simulink library "rewardLibrary"  (R2022b)
settings: Solver=VariableStepAuto  StartTime=0.0  StopTime=10.0  RelTol=1e-3
values from neighbouring files (symbols this model uses):
  accel_vec = (-4:0.5:4)'    [setUpModel.m]
  Ts = 0.1    [setUpMPC.m]
  TsRL = Ts    [setUpRLEnv.m]
  vel_vec = 0:2:20    [setUpModel.m]
undefined symbols (not defined in the file or in its folder): A, B, C, curvature1, D, D_default, DiscIntNeverNeededParam, E, F, gradbp1, k_sigmoid, steer_lim, t_gap, v_set, x_colpen, y_colpen, Z_colpen
libraries: simulink x379, $bdroot x2, mpcadaslib x1
(part 8 of 9)

== system rewardLibrary/Obs // Reward 8-7/Path following ==
  v_err : Inport
  e1 : Inport  Port=2
  e2 : Inport  Port=3
  steer : Inport  Port=4
  accel : Inport  Port=5
  Exp{,1..4} (5 alike) : Math
  Gain1 : Gain  Gain=0.5
  Gain11 : Gain  Gain=-0.1
  Gain12 : Gain  Gain=1.5
  Gain2 : Gain  Gain=0.2
  Gain3 : Gain  Gain=0.1
  Gain4 : Gain  Gain=-0.5
  Gain5 : Gain  Gain=-10
  Gain6 : Gain  Gain=1.5
  Gain8 : Gain  Gain=-0.1
  Gain9 : Gain  Gain=-0.125
  Math Function2 : Math  Operator=square  SignedPower=on
  Square{1..4} (4 alike) : Math  Operator=square  SignedPower=on
  Sum1 : Sum  Inputs=+++++
  Unit Delay : UnitDelay  SampleTime=-1  HasFrameUpgradeWarning=on
  Unit Delay1 : UnitDelay  SampleTime=-1  HasFrameUpgradeWarning=on
  r_pf : Outport  VectorParamsAs1DForOutWhenUnconnected=off
  wires:
  Gain12/1 -> Sum1/1
  Gain6/1 -> Sum1/2
  Gain1/1 -> Sum1/3
  Gain2/1 -> Sum1/4
  Gain3/1 -> Sum1/5
  Exp4/1 -> Gain3/1
  Exp3/1 -> Gain2/1
  Exp2/1 -> Gain1/1
  Exp1/1 -> Gain6/1
  Gain9/1 -> Exp1/1
  Gain4/1 -> Exp2/1
  Gain5/1 -> Exp3/1
  Gain8/1 -> Exp4/1
  Square1/1 -> Gain9/1
  Math Function2/1 -> Gain5/1
  Square3/1 -> Gain8/1
  Unit Delay1/1 -> Square3/1
  Unit Delay/1 -> Math Function2/1  "u_prev"
  e2/1 -> Square2/1
  e1/1 -> Square1/1
  steer/1 -> Unit Delay/1
  Square2/1 -> Gain4/1
  accel/1 -> Unit Delay1/1
  Sum1/1 -> r_pf/1
  v_err/1 -> Square4/1
  Exp/1 -> Gain12/1
  Square4/1 -> Gain11/1
  Gain11/1 -> Exp/1

== system rewardLibrary/Obs // Reward 8-7/Subsystem ==
  v_ego : Inport
  v_ref : Inport  Port=2
  e1 : Inport  Port=3
  e2 : Inport  Port=4
  e1dot : Inport  Port=5
  e2dot : Inport  Port=6
  v_lead : Inport  Port=7
  xgap : Inport  Port=8
  ygap : Inport  Port=9
  Add : Sum  Inputs=+-
  Discrete-Time Integrator1 : DiscreteIntegrator  SampleTime=-1  ICPrevOutput=DiscIntNeverNeededParam  ICPrevScaledInput=DiscIntNeverNeededParam
  Discrete-Time Integrator2 : DiscreteIntegrator  SampleTime=-1  ICPrevOutput=DiscIntNeverNeededParam  ICPrevScaledInput=DiscIntNeverNeededParam
  Discrete-Time Integrator3 : DiscreteIntegrator  SampleTime=-1  ICPrevOutput=DiscIntNeverNeededParam  ICPrevScaledInput=DiscIntNeverNeededParam
  Lateral deviation : Scope
  Mux : Mux  Inputs=12
  obs : Outport  VectorParamsAs1DForOutWhenUnconnected=off
  v_err : Outport  Port=2  VectorParamsAs1DForOutWhenUnconnected=off
  wires:
  v_ref/1 -> Add/1  "d_rel"
  e2dot/1 -> Mux/9
  e1dot/1 -> Mux/8
  Mux/1 -> obs/1
  Discrete-Time Integrator2/1 -> Mux/4  "integral_error"
  e2/1 -> Discrete-Time Integrator3/1, Mux/7
  Discrete-Time Integrator1/1 -> Mux/1  "integral_error"
  e1/1 -> Discrete-Time Integrator2/1, Mux/5, Lateral deviation/1
  v_ego/1 -> Mux/3, Add/2
  Discrete-Time Integrator3/1 -> Mux/6  "integral_error"
  Add/1 -> Discrete-Time Integrator1/1, Mux/2, v_err/1
  v_lead/1 -> Mux/10
  xgap/1 -> Mux/11
  ygap/1 -> Mux/12

== system rewardLibrary/Obs // Reward 8-7/Subsystem2 ==
  v_ego : Inport
  e1 : Inport  Port=2
  e2 : Inport  Port=3
  xgap : Inport  Port=4
  collided : Inport  Port=5
  AND : Logic  IconShape=distinctive  AllPortsSameDT=off  OutDataTypeStr=boolean
  AND1 : Logic  IconShape=distinctive  AllPortsSameDT=off  OutDataTypeStr=boolean
  Abs : Abs  SaturateOnIntegerOverflow=off
  Abs1 : Abs  SaturateOnIntegerOverflow=off
  Compare To Constant : simulink/Logic and Bit Operations/Compare To Constant  relop=>  const=90  OutDataTypeStr=boolean
  Compare To Constant1 : simulink/Logic and Bit Operations/Compare To Constant  relop=>  const=0  OutDataTypeStr=boolean
  Constant : Constant
  Constant3 : Constant  Value=0
  Demux : Demux  Outputs=2
  Detect Rise Positive : simulink/Logic and Bit Operations/Detect Rise Positive  vinit=0  OutDataTypeStr=boolean
  Lateral deviation : simulink/Logic and Bit Operations/Compare To Constant  relop=>  const=8  OutDataTypeStr=boolean
  Logical Operator1 : Logic  Operator=OR  Inputs=3  AllPortsSameDT=off  OutDataTypeStr=boolean
  R2D : Gain  Gain=180/pi
  Relative yaw angle : simulink/Logic and Bit Operations/Compare To Constant  relop=>  const=55  OutDataTypeStr=boolean
  Switch : Switch  Criteria=u2 > Threshold  Threshold=90  SaturateOnIntegerOverflow=off  InputSameDT=off
  Terminator : Terminator
  Velocity : simulink/Logic and Bit Operations/Compare To Constant  relop=<  const=2  OutDataTypeStr=boolean
  Velocity1 : simulink/Logic and Bit Operations/Compare To Constant  relop=<  const=10  OutDataTypeStr=boolean
  fail : Outport  VectorParamsAs1DForOutWhenUnconnected=off
  failCollided : Outport  Port=2  VectorParamsAs1DForOutWhenUnconnected=off
  completeCourse : Outport  Port=3  VectorParamsAs1DForOutWhenUnconnected=off
  overtakeSuccess : Outport  Port=4  VectorParamsAs1DForOutWhenUnconnected=off
  wires:
  Demux/2 -> Compare To Constant/1, Switch/2  "y2"
  [pos2] -> Demux/1
  Demux/1 -> Terminator/1
  Logical Operator1/1 -> fail/1
  Constant3/1 -> Switch/3
  Constant/1 -> Switch/1
  Switch/1 -> completeCourse/1
  AND/1 -> Logical Operator1/3  "spinTurn"
  Relative yaw angle/1 -> AND/2
  R2D/1 -> Relative yaw angle/1
  Abs1/1 -> R2D/1
  e2/1 -> Abs1/1
  Velocity1/1 -> AND/1
  e1/1 -> Abs/1
  Abs/1 -> Lateral deviation/1
  v_ego/1 -> Velocity/1, Velocity1/1
  Lateral deviation/1 -> Logical Operator1/2
  Velocity/1 -> Logical Operator1/1  "tooSlow"
  Compare To Constant/1 -> Detect Rise Positive/1
  Detect Rise Positive/1 -> AND1/1
  xgap/1 -> Compare To Constant1/1
  Compare To Constant1/1 -> AND1/2
  AND1/1 -> overtakeSuccess/1
  collided/1 -> failCollided/1

== system rewardLibrary/Obs // Reward 8-9/Overtaking ==
  ry : Inport
  G : Inport  Port=2
  Add : Sum  Inputs=+-
  Compare To Constant : simulink/Logic and Bit Operations/Compare To Constant  Commented=on  relop=>  const=0  OutDataTypeStr=boolean
  Constant : Constant
  Constant1 : Constant  Value=0
  D : Gain  Gain=2
  F : Gain  Commented=on  Gain=3
  Gain1 : Gain  Gain=2
  Gain6 : Gain  Gain=0.75
  Sigmoid : Subsystem
  Slipstream reward enable : Switch  Criteria=u2 > Threshold  Threshold=-5  SaturateOnIntegerOverflow=off  InputSameDT=off
  Sum1 : Sum  Inputs=+++
  r_ot : Outport  VectorParamsAs1DForOutWhenUnconnected=off
  wires:
  Compare To Constant/1 -> F/1
  F/1 -> Sum1/3
  Constant1/1 -> Slipstream reward enable/1
  Gain6/1 -> Slipstream reward enable/3
  G/1 -> Sigmoid/1(x), Slipstream reward enable/2, Compare To Constant/1
  Add/1 -> D/1
  D/1 -> Sum1/2
  Constant/1 -> Add/2
  Gain1/1 -> Add/1
  Sigmoid/1(sigmoid) -> Gain1/1
  ry/1 -> Gain6/1
  Slipstream reward enable/1 -> Sum1/1
  Sum1/1 -> r_ot/1

== system rewardLibrary/Obs // Reward 8-9/Path following ==
  v_err : Inport
  e1 : Inport  Port=2
  e2 : Inport  Port=3
  steer : Inport  Port=4
  accel : Inport  Port=5
  Exp{,1..4} (5 alike) : Math
  Gain1 : Gain  Gain=0.5
  Gain11 : Gain  Gain=-0.006
  Gain12 : Gain  Gain=4
  Gain2 : Gain  Gain=0.2
  Gain3 : Gain  Gain=0.1
  Gain4 : Gain  Gain=-0.9
  Gain5 : Gain  Gain=-10
  Gain6 : Gain  Gain=1.5
  Gain8 : Gain  Gain=-0.1
  Gain9 : Gain  Gain=-0.125
  Math Function2 : Math  Operator=square  SignedPower=on
  Square{1..4} (4 alike) : Math  Operator=square  SignedPower=on
  Sum1 : Sum  Inputs=+++++
  Unit Delay : UnitDelay  SampleTime=-1  HasFrameUpgradeWarning=on
  Unit Delay1 : UnitDelay  SampleTime=-1  HasFrameUpgradeWarning=on
  r_pf : Outport  VectorParamsAs1DForOutWhenUnconnected=off
  wires:
  Gain11/1 -> Exp/1
  Square4/1 -> Gain11/1
  Exp/1 -> Gain12/1
  v_err/1 -> Square4/1
  Sum1/1 -> r_pf/1
  accel/1 -> Unit Delay1/1
  Square2/1 -> Gain4/1
  steer/1 -> Unit Delay/1
  e1/1 -> Square1/1
  e2/1 -> Square2/1
  Unit Delay/1 -> Math Function2/1  "u_prev"
  Unit Delay1/1 -> Square3/1
  Square3/1 -> Gain8/1
  Math Function2/1 -> Gain5/1
  Square1/1 -> Gain9/1
  Gain8/1 -> Exp4/1
  Gain5/1 -> Exp3/1
  Gain4/1 -> Exp2/1
  Gain9/1 -> Exp1/1
  Exp1/1 -> Gain6/1
  Exp2/1 -> Gain1/1
  Exp3/1 -> Gain2/1
  Exp4/1 -> Gain3/1
  Gain3/1 -> Sum1/5
  Gain2/1 -> Sum1/4
  Gain1/1 -> Sum1/3
  Gain6/1 -> Sum1/2
  Gain12/1 -> Sum1/1

== system rewardLibrary/Obs // Reward 8-9/Subsystem ==
  v_ego : Inport
  v_ref : Inport  Port=2
  e1 : Inport  Port=3
  e2 : Inport  Port=4
  e1dot : Inport  Port=5
  e2dot : Inport  Port=6
  v_lead : Inport  Port=7
  xgap : Inport  Port=8
  ygap : Inport  Port=9
  Add : Sum  Inputs=+-
  Discrete-Time Integrator1 : DiscreteIntegrator  SampleTime=-1  ICPrevOutput=DiscIntNeverNeededParam  ICPrevScaledInput=DiscIntNeverNeededParam
  Discrete-Time Integrator2 : DiscreteIntegrator  SampleTime=-1  ICPrevOutput=DiscIntNeverNeededParam  ICPrevScaledInput=DiscIntNeverNeededParam
  Discrete-Time Integrator3 : DiscreteIntegrator  SampleTime=-1  ICPrevOutput=DiscIntNeverNeededParam  ICPrevScaledInput=DiscIntNeverNeededParam
  Lateral deviation : Scope
  Mux : Mux  Inputs=12
  obs : Outport  VectorParamsAs1DForOutWhenUnconnected=off
  v_err : Outport  Port=2  VectorParamsAs1DForOutWhenUnconnected=off
  wires:
  ygap/1 -> Mux/12
  xgap/1 -> Mux/11
  v_lead/1 -> Mux/10
  Add/1 -> v_err/1, Mux/2, Discrete-Time Integrator1/1
  Discrete-Time Integrator3/1 -> Mux/6  "integral_error"
  v_ego/1 -> Add/2, Mux/3
  e1/1 -> Lateral deviation/1, Mux/5, Discrete-Time Integrator2/1
  Discrete-Time Integrator1/1 -> Mux/1  "integral_error"
  e2/1 -> Mux/7, Discrete-Time Integrator3/1
  Discrete-Time Integrator2/1 -> Mux/4  "integral_error"
  Mux/1 -> obs/1
  e1dot/1 -> Mux/8
  e2dot/1 -> Mux/9
  v_ref/1 -> Add/1  "d_rel"

== system rewardLibrary/Obs // Reward 8-9/Subsystem2 ==
  v_ego : Inport
  e1 : Inport  Port=2
  e2 : Inport  Port=3
  xgap : Inport  Port=4
  collided : Inport  Port=5
  AND : Logic  IconShape=distinctive  AllPortsSameDT=off  OutDataTypeStr=boolean
  AND1 : Logic  IconShape=distinctive  AllPortsSameDT=off  OutDataTypeStr=boolean
  Abs : Abs  SaturateOnIntegerOverflow=off
  Abs1 : Abs  SaturateOnIntegerOverflow=off
  Compare To Constant : simulink/Logic and Bit Operations/Compare To Constant  relop=>  const=90  OutDataTypeStr=boolean
  Compare To Constant1 : simulink/Logic and Bit Operations/Compare To Constant  relop=>  const=0  OutDataTypeStr=boolean
  Constant : Constant
  Constant3 : Constant  Value=0
  Demux : Demux  Outputs=2
  Detect Rise Positive : simulink/Logic and Bit Operations/Detect Rise Positive  vinit=0  OutDataTypeStr=boolean
  Lateral deviation : simulink/Logic and Bit Operations/Compare To Constant  relop=>  const=8  OutDataTypeStr=boolean
  Logical Operator1 : Logic  Operator=OR  Inputs=3  AllPortsSameDT=off  OutDataTypeStr=boolean
  R2D : Gain  Gain=180/pi
  Relative yaw angle : simulink/Logic and Bit Operations/Compare To Constant  relop=>  const=55  OutDataTypeStr=boolean
  Switch : Switch  Criteria=u2 > Threshold  Threshold=90  SaturateOnIntegerOverflow=off  InputSameDT=off
  Terminator : Terminator
  Velocity : simulink/Logic and Bit Operations/Compare To Constant  relop=<  const=2  OutDataTypeStr=boolean
  Velocity1 : simulink/Logic and Bit Operations/Compare To Constant  relop=<  const=10  OutDataTypeStr=boolean
  fail : Outport  VectorParamsAs1DForOutWhenUnconnected=off
  failCollided : Outport  Port=2  VectorParamsAs1DForOutWhenUnconnected=off
  completeCourse : Outport  Port=3  VectorParamsAs1DForOutWhenUnconnected=off
  overtakeSuccess : Outport  Port=4  VectorParamsAs1DForOutWhenUnconnected=off
  wires:
  collided/1 -> failCollided/1
  AND1/1 -> overtakeSuccess/1
  Compare To Constant1/1 -> AND1/2
  xgap/1 -> Compare To Constant1/1
  Detect Rise Positive/1 -> AND1/1
  Compare To Constant/1 -> Detect Rise Positive/1
  Velocity/1 -> Logical Operator1/1  "tooSlow"
  Lateral deviation/1 -> Logical Operator1/2
  v_ego/1 -> Velocity1/1, Velocity/1
  Abs/1 -> Lateral deviation/1
  e1/1 -> Abs/1
  Velocity1/1 -> AND/1
  e2/1 -> Abs1/1
  Abs1/1 -> R2D/1
  R2D/1 -> Relative yaw angle/1
  Relative yaw angle/1 -> AND/2
  AND/1 -> Logical Operator1/3  "spinTurn"
  Switch/1 -> completeCourse/1
  Constant/1 -> Switch/1
  Constant3/1 -> Switch/3
  Logical Operator1/1 -> fail/1
  Demux/1 -> Terminator/1
  [pos2] -> Demux/1
  Demux/2 -> Switch/2, Compare To Constant/1  "y2"

== system rewardLibrary/Obs // Reward 9-1/Overtaking ==
  note: lead
  ry : Inport
  G : Inport  Port=2
  -k : Gain  Gain=-0.4
  Add : Sum
  Add1 : Sum  Inputs=+-
  C : Gain  Gain=0
  Constant : Constant
  Constant1 : Constant  Value=0
  Constant2 : Constant
  D : Gain  Gain=3
  Divide : Product  Inputs=*/
  Exp : Math
  Slipstream reward enable : Switch  Criteria=u2 > Threshold  Threshold=-6.5  SaturateOnIntegerOverflow=off  InputSameDT=off
  Sum1 : Sum
  h : Constant  Value=-2
  r_ot : Outport  VectorParamsAs1DForOutWhenUnconnected=off
  wires:
  Constant1/1 -> Slipstream reward enable/1
  C/1 -> Slipstream reward enable/3
  Divide/1 -> D/1
  ry/1 -> C/1
  Slipstream reward enable/1 -> Sum1/1
  Sum1/1 -> r_ot/1
  D/1 -> Sum1/2
  Exp/1 -> Add/1
  G/1 -> Add1/1, Slipstream reward enable/2
  Constant/1 -> Divide/1
  -k/1 -> Exp/1
  Constant2/1 -> Add/2
  Add/1 -> Divide/2
  Add1/1 -> -k/1
  h/1 -> Add1/2

== system rewardLibrary/Obs // Reward 9-1/Path following ==
  v_err : Inport
  e1 : Inport  Port=2
  e2 : Inport  Port=3
  steer : Inport  Port=4
  accel : Inport  Port=5
  Constant : Constant  Value=0.5
  Exp{,1..4} (5 alike) : Math
  Gain1 : Gain  Gain=0.5
  Gain11 : Gain  Gain=-0.15
  Gain12 : Gain
  Gain2 : Gain  Gain=0.2
  Gain3 : Gain  Gain=0.1
  Gain4 : Gain  Gain=-0.9
  Gain5 : Gain  Gain=-10
  Gain6 : Gain  Gain=1.5
  Gain8 : Gain  Gain=-0.1
  Gain9 : Gain  Gain=-0.06
  Math Function2 : Math  Operator=square  SignedPower=on
  Square{1..4} (4 alike) : Math  Operator=square  SignedPower=on
  Sum1 : Sum  Inputs=++++++
  Unit Delay : UnitDelay  SampleTime=-1  HasFrameUpgradeWarning=on
  Unit Delay1 : UnitDelay  SampleTime=-1  HasFrameUpgradeWarning=on
  r_pf : Outport  VectorParamsAs1DForOutWhenUnconnected=off
  wires:
  Gain11/1 -> Exp/1
  Square4/1 -> Gain11/1
  Exp/1 -> Gain12/1
  v_err/1 -> Square4/1
  Sum1/1 -> r_pf/1
  accel/1 -> Unit Delay1/1
  Square2/1 -> Gain4/1
  steer/1 -> Unit Delay/1
  e1/1 -> Square1/1
  e2/1 -> Square2/1
  Unit Delay/1 -> Math Function2/1  "u_prev"
  Unit Delay1/1 -> Square3/1
  Square3/1 -> Gain8/1
  Math Function2/1 -> Gain5/1
  Square1/1 -> Gain9/1
  Gain8/1 -> Exp4/1
  Gain5/1 -> Exp3/1
  Gain4/1 -> Exp2/1
  Gain9/1 -> Exp1/1
  Exp1/1 -> Gain6/1
  Exp2/1 -> Gain1/1
  Exp3/1 -> Gain2/1
  Exp4/1 -> Gain3/1
  Gain3/1 -> Sum1/5
  Gain2/1 -> Sum1/4
  Gain1/1 -> Sum1/3
  Gain6/1 -> Sum1/2
  Gain12/1 -> Sum1/1
  Constant/1 -> Sum1/6

== system rewardLibrary/Obs // Reward 9-1/Subsystem ==
  v_ego : Inport
  v_ref : Inport  Port=2
  e1 : Inport  Port=3
  e2 : Inport  Port=4
  e1dot : Inport  Port=5
  e2dot : Inport  Port=6
  v_lead : Inport  Port=7
  xgap : Inport  Port=8
  ygap : Inport  Port=9
  Add : Sum  Inputs=+-
  Discrete-Time Integrator1 : DiscreteIntegrator  SampleTime=-1  ICPrevOutput=DiscIntNeverNeededParam  ICPrevScaledInput=DiscIntNeverNeededParam
  Discrete-Time Integrator2 : DiscreteIntegrator  SampleTime=-1  ICPrevOutput=DiscIntNeverNeededParam  ICPrevScaledInput=DiscIntNeverNeededParam
  Discrete-Time Integrator3 : DiscreteIntegrator  SampleTime=-1  ICPrevOutput=DiscIntNeverNeededParam  ICPrevScaledInput=DiscIntNeverNeededParam
  Lateral deviation : Scope
  Mux : Mux  Inputs=12
  obs : Outport  VectorParamsAs1DForOutWhenUnconnected=off
  v_err : Outport  Port=2  VectorParamsAs1DForOutWhenUnconnected=off
  wires:
  ygap/1 -> Mux/12
  xgap/1 -> Mux/11
  v_lead/1 -> Mux/10
  Add/1 -> v_err/1, Mux/2, Discrete-Time Integrator1/1
  Discrete-Time Integrator3/1 -> Mux/6  "integral_error"
  v_ego/1 -> Add/2, Mux/3
  e1/1 -> Lateral deviation/1, Mux/5, Discrete-Time Integrator2/1
  Discrete-Time Integrator1/1 -> Mux/1  "integral_error"
  e2/1 -> Mux/7, Discrete-Time Integrator3/1
  Discrete-Time Integrator2/1 -> Mux/4  "integral_error"
  Mux/1 -> obs/1
  e1dot/1 -> Mux/8
  e2dot/1 -> Mux/9
  v_ref/1 -> Add/1  "d_rel"

== system rewardLibrary/Obs // Reward 9-1/Subsystem2 ==
  v_ego : Inport
  e1 : Inport  Port=2
  e2 : Inport  Port=3
  xgap : Inport  Port=4
  collided : Inport  Port=5
  AND : Logic  IconShape=distinctive  AllPortsSameDT=off  OutDataTypeStr=boolean
  AND1 : Logic  IconShape=distinctive  AllPortsSameDT=off  OutDataTypeStr=boolean
  Abs : Abs  SaturateOnIntegerOverflow=off
  Abs1 : Abs  SaturateOnIntegerOverflow=off
  Compare To Constant : simulink/Logic and Bit Operations/Compare To Constant  relop=>  const=90  OutDataTypeStr=boolean
  Compare To Constant1 : simulink/Logic and Bit Operations/Compare To Constant  relop=>  const=0  OutDataTypeStr=boolean
  Constant : Constant
  Constant3 : Constant  Value=0
  Demux : Demux  Outputs=2
  Detect Rise Positive : simulink/Logic and Bit Operations/Detect Rise Positive  vinit=0  OutDataTypeStr=boolean
  Lateral deviation : simulink/Logic and Bit Operations/Compare To Constant  relop=>  const=8  OutDataTypeStr=boolean
  Logical Operator1 : Logic  Operator=OR  Inputs=3  AllPortsSameDT=off  OutDataTypeStr=boolean
  R2D : Gain  Gain=180/pi
  Relative yaw angle : simulink/Logic and Bit Operations/Compare To Constant  relop=>  const=40  OutDataTypeStr=boolean
  Switch : Switch  Criteria=u2 > Threshold  Threshold=90  SaturateOnIntegerOverflow=off  InputSameDT=off
  Terminator : Terminator
  Velocity : simulink/Logic and Bit Operations/Compare To Constant  relop=<  const=2  OutDataTypeStr=boolean
  Velocity1 : simulink/Logic and Bit Operations/Compare To Constant  relop=<  const=10  OutDataTypeStr=boolean
  fail : Outport  VectorParamsAs1DForOutWhenUnconnected=off
  failCollided : Outport  Port=2  VectorParamsAs1DForOutWhenUnconnected=off
  completeCourse : Outport  Port=3  VectorParamsAs1DForOutWhenUnconnected=off
  overtakeSuccess : Outport  Port=4  VectorParamsAs1DForOutWhenUnconnected=off
  wires:
  collided/1 -> failCollided/1
  AND1/1 -> overtakeSuccess/1
  Compare To Constant1/1 -> AND1/2
  xgap/1 -> Compare To Constant1/1
  Detect Rise Positive/1 -> AND1/1
  Compare To Constant/1 -> Detect Rise Positive/1
  Velocity/1 -> Logical Operator1/1  "tooSlow"
  Lateral deviation/1 -> Logical Operator1/2
  v_ego/1 -> Velocity1/1, Velocity/1
  Abs/1 -> Lateral deviation/1
  e1/1 -> Abs/1
  Velocity1/1 -> AND/1
  e2/1 -> Abs1/1
  Abs1/1 -> R2D/1
  R2D/1 -> Relative yaw angle/1
  Relative yaw angle/1 -> AND/2
  AND/1 -> Logical Operator1/3  "spinTurn"
  Switch/1 -> completeCourse/1
  Constant/1 -> Switch/1
  Constant3/1 -> Switch/3
  Logical Operator1/1 -> fail/1
  Demux/1 -> Terminator/1
  [pos2] -> Demux/1
  Demux/2 -> Switch/2, Compare To Constant/1  "y2"

== system rewardLibrary/Obs // Reward 9-2/Overtaking ==
  note: Overtake on right sigmoid
  note: Overtaking reward sigmoid
  ry : Inport
  xgap : Inport  Port=2
  ygap : Inport  Port=3
  -k : Gain  Gain=-0.4
  -k1 : Gain  Gain=-3
  Add : Sum
  Add1 : Sum  Inputs=+-
  Add2 : Sum
  C : Gain  Gain=0
  Constant{,2..4} (4 alike) : Constant
  Constant1 : Constant  Value=0
  Constant5 : Constant  Value=0
  D : Gain  Gain=3
  Divide : Product  Inputs=*/
  Divide1 : Product  Inputs=*/
  Exp : Math
  Exp1 : Math
  G : Gain
  Slipstream reward enable : Switch  Criteria=u2 > Threshold  Threshold=-6.5  SaturateOnIntegerOverflow=off  InputSameDT=off
  Slipstream reward enable1 : Switch  Criteria=u2 > Threshold  SaturateOnIntegerOverflow=off  InputSameDT=off
  Sum1 : Sum  Inputs=+++
  h : Constant  Value=-2
  r_ot : Outport  VectorParamsAs1DForOutWhenUnconnected=off
  wires:
  Constant1/1 -> Slipstream reward enable/1
  C/1 -> Slipstream reward enable/3
  Divide/1 -> D/1
  ry/1 -> C/1
  Slipstream reward enable/1 -> Sum1/1
  Sum1/1 -> r_ot/1
  D/1 -> Sum1/2
  Exp/1 -> Add/1
  xgap/1 -> Slipstream reward enable/2, Slipstream reward enable1/2, Add1/1
  Constant/1 -> Divide/1
  -k/1 -> Exp/1
  Constant2/1 -> Add/2
  Add/1 -> Divide/2
  Add1/1 -> -k/1
  h/1 -> Add1/2
  Constant4/1 -> Add2/2
  Add2/1 -> Divide1/2
  -k1/1 -> Exp1/1
  Exp1/1 -> Add2/1
  Constant3/1 -> Divide1/1
  Divide1/1 -> G/1
  G/1 -> Sum1/3
  ygap/1 -> Slipstream reward enable1/3
  Constant5/1 -> Slipstream reward enable1/1
  Slipstream reward enable1/1 -> -k1/1

== system rewardLibrary/Obs // Reward 9-2/Path following ==
  v_err : Inport
  e1 : Inport  Port=2
  e2 : Inport  Port=3
  steer : Inport  Port=4
  accel : Inport  Port=5
  Constant : Constant  Commented=on  Value=0.5
  Exp{,1..4} (5 alike) : Math
  Gain1 : Gain  Gain=0.5
  Gain11 : Gain  Gain=-0.15
  Gain12 : Gain
  Gain2 : Gain  Gain=0.2
  Gain3 : Gain  Gain=0.1
  Gain4 : Gain  Gain=-0.9
  Gain5 : Gain  Gain=-10
  Gain6 : Gain  Gain=1.5
  Gain8 : Gain  Gain=-0.1
  Gain9 : Gain  Gain=-0.06
  Math Function2 : Math  Operator=square  SignedPower=on
  Square{1..4} (4 alike) : Math  Operator=square  SignedPower=on
  Sum1 : Sum  Inputs=++++++
  Unit Delay : UnitDelay  SampleTime=-1  HasFrameUpgradeWarning=on
  Unit Delay1 : UnitDelay  SampleTime=-1  HasFrameUpgradeWarning=on
  r_pf : Outport  VectorParamsAs1DForOutWhenUnconnected=off
  wires:
  Gain11/1 -> Exp/1
  Square4/1 -> Gain11/1
  Exp/1 -> Gain12/1
  v_err/1 -> Square4/1
  Sum1/1 -> r_pf/1
  accel/1 -> Unit Delay1/1
  Square2/1 -> Gain4/1
  steer/1 -> Unit Delay/1
  e1/1 -> Square1/1
  e2/1 -> Square2/1
  Unit Delay/1 -> Math Function2/1  "u_prev"
  Unit Delay1/1 -> Square3/1
  Square3/1 -> Gain8/1
  Math Function2/1 -> Gain5/1
  Square1/1 -> Gain9/1
  Gain8/1 -> Exp4/1
  Gain5/1 -> Exp3/1
  Gain4/1 -> Exp2/1
  Gain9/1 -> Exp1/1
  Exp1/1 -> Gain6/1
  Exp2/1 -> Gain1/1
  Exp3/1 -> Gain2/1
  Exp4/1 -> Gain3/1
  Gain3/1 -> Sum1/5
  Gain2/1 -> Sum1/4
  Gain1/1 -> Sum1/3
  Gain6/1 -> Sum1/2
  Gain12/1 -> Sum1/1
  Constant/1 -> Sum1/6

== system rewardLibrary/Obs // Reward 9-2/Subsystem ==
  v_ego : Inport
  v_ref : Inport  Port=2
  e1 : Inport  Port=3
  e2 : Inport  Port=4
  e1dot : Inport  Port=5
  e2dot : Inport  Port=6
  v_lead : Inport  Port=7
  xgap : Inport  Port=8
  ygap : Inport  Port=9
  Add : Sum  Inputs=+-
  Discrete-Time Integrator1 : DiscreteIntegrator  SampleTime=-1  ICPrevOutput=DiscIntNeverNeededParam  ICPrevScaledInput=DiscIntNeverNeededParam
  Discrete-Time Integrator2 : DiscreteIntegrator  SampleTime=-1  ICPrevOutput=DiscIntNeverNeededParam  ICPrevScaledInput=DiscIntNeverNeededParam
  Discrete-Time Integrator3 : DiscreteIntegrator  SampleTime=-1  ICPrevOutput=DiscIntNeverNeededParam  ICPrevScaledInput=DiscIntNeverNeededParam
  Lateral deviation : Scope
  Mux : Mux  Inputs=12
  obs : Outport  VectorParamsAs1DForOutWhenUnconnected=off
  v_err : Outport  Port=2  VectorParamsAs1DForOutWhenUnconnected=off
  wires:
  ygap/1 -> Mux/12
  xgap/1 -> Mux/11
  v_lead/1 -> Mux/10
  Add/1 -> v_err/1, Mux/2, Discrete-Time Integrator1/1
  Discrete-Time Integrator3/1 -> Mux/6  "integral_error"
  v_ego/1 -> Add/2, Mux/3
  e1/1 -> Lateral deviation/1, Mux/5, Discrete-Time Integrator2/1
  Discrete-Time Integrator1/1 -> Mux/1  "integral_error"
  e2/1 -> Mux/7, Discrete-Time Integrator3/1
  Discrete-Time Integrator2/1 -> Mux/4  "integral_error"
  Mux/1 -> obs/1
  e1dot/1 -> Mux/8
  e2dot/1 -> Mux/9
  v_ref/1 -> Add/1  "d_rel"

== system rewardLibrary/Obs // Reward 9-2/Subsystem2 ==
  v_ego : Inport
  e1 : Inport  Port=2
  e2 : Inport  Port=3
  xgap : Inport  Port=4
  collided : Inport  Port=5
  AND : Logic  IconShape=distinctive  AllPortsSameDT=off  OutDataTypeStr=boolean
  AND1 : Logic  IconShape=distinctive  AllPortsSameDT=off  OutDataTypeStr=boolean
  Abs : Abs  SaturateOnIntegerOverflow=off
  Abs1 : Abs  SaturateOnIntegerOverflow=off
  Compare To Constant : simulink/Logic and Bit Operations/Compare To Constant  relop=>  const=90  OutDataTypeStr=boolean
  Compare To Constant1 : simulink/Logic and Bit Operations/Compare To Constant  relop=>  const=0  OutDataTypeStr=boolean
  Constant : Constant
  Constant3 : Constant  Value=0
  Demux : Demux  Outputs=2
  Detect Rise Positive : simulink/Logic and Bit Operations/Detect Rise Positive  vinit=0  OutDataTypeStr=boolean
  Lateral deviation : simulink/Logic and Bit Operations/Compare To Constant  relop=>  const=8  OutDataTypeStr=boolean
  Logical Operator1 : Logic  Operator=OR  Inputs=3  AllPortsSameDT=off  OutDataTypeStr=boolean
  R2D : Gain  Gain=180/pi
  Relative yaw angle : simulink/Logic and Bit Operations/Compare To Constant  relop=>  const=40  OutDataTypeStr=boolean
  Switch : Switch  Criteria=u2 > Threshold  Threshold=90  SaturateOnIntegerOverflow=off  InputSameDT=off
  Terminator : Terminator
  Velocity : simulink/Logic and Bit Operations/Compare To Constant  relop=<  const=2  OutDataTypeStr=boolean
  Velocity1 : simulink/Logic and Bit Operations/Compare To Constant  relop=<  const=10  OutDataTypeStr=boolean
  fail : Outport  VectorParamsAs1DForOutWhenUnconnected=off
  failCollided : Outport  Port=2  VectorParamsAs1DForOutWhenUnconnected=off
  completeCourse : Outport  Port=3  VectorParamsAs1DForOutWhenUnconnected=off
  overtakeSuccess : Outport  Port=4  VectorParamsAs1DForOutWhenUnconnected=off
  wires:
  collided/1 -> failCollided/1
  AND1/1 -> overtakeSuccess/1
  Compare To Constant1/1 -> AND1/2
  xgap/1 -> Compare To Constant1/1
  Detect Rise Positive/1 -> AND1/1
  Compare To Constant/1 -> Detect Rise Positive/1
  Velocity/1 -> Logical Operator1/1  "tooSlow"
  Lateral deviation/1 -> Logical Operator1/2
  v_ego/1 -> Velocity1/1, Velocity/1
  Abs/1 -> Lateral deviation/1
  e1/1 -> Abs/1
  Velocity1/1 -> AND/1
  e2/1 -> Abs1/1
  Abs1/1 -> R2D/1
  R2D/1 -> Relative yaw angle/1
  Relative yaw angle/1 -> AND/2
  AND/1 -> Logical Operator1/3  "spinTurn"
  Switch/1 -> completeCourse/1
  Constant/1 -> Switch/1
  Constant3/1 -> Switch/3
  Logical Operator1/1 -> fail/1
  Demux/1 -> Terminator/1
  [pos2] -> Demux/1
  Demux/2 -> Switch/2, Compare To Constant/1  "y2"

== system rewardLibrary/Obs // Reward 9-3/Overtaking ==
  note: Overtake on right sigmoid
  note: Overtaking reward sigmoid
  ry : Inport
  xgap : Inport  Port=2
  ygap : Inport  Port=3
  -k_D : Gain  Gain=-0.4
  -k_G : Gain  Gain=-1.2
  Add : Sum
  Add1 : Sum  Inputs=+-
  Add2 : Sum
  C : Gain  Gain=0
  Constant{,2..4} (4 alike) : Constant
  Constant1 : Constant  Value=0
  D : Gain  Gain=3
  Divide : Product  Inputs=*/
  Divide1 : Product  Inputs=*/
  Exp : Math
  Exp1 : Math
  G : Gain  Gain=0.5
  G1 : Constant  Value=0.5
  Memory : Memory
  Slipstream reward enable : Switch  Criteria=u2 > Threshold  Threshold=-6.5  SaturateOnIntegerOverflow=off  InputSameDT=off
  Subsystem : Subsystem  Commented=on
  Sum1 : Sum  Inputs=+++
  h : Constant  Value=-2
  switch2 : Switch  Criteria=u2 > Threshold  SaturateOnIntegerOverflow=off  InputSameDT=off
  r_ot : Outport  VectorParamsAs1DForOutWhenUnconnected=off
  wires:
  Constant1/1 -> Slipstream reward enable/1
  C/1 -> Slipstream reward enable/3
  Divide/1 -> D/1
  ry/1 -> C/1
  Slipstream reward enable/1 -> Sum1/1
  Sum1/1 -> r_ot/1
  D/1 -> Sum1/2
  Exp/1 -> Add/1
  Constant/1 -> Divide/1
  -k_D/1 -> Exp/1
  Constant2/1 -> Add/2
  Add/1 -> Divide/2
  Add1/1 -> -k_D/1
  h/1 -> Add1/2
  Constant4/1 -> Add2/2
  Add2/1 -> Divide1/2
  -k_G/1 -> Exp1/1
  Exp1/1 -> Add2/1
  Constant3/1 -> Divide1/1
  Divide1/1 -> G/1
  ygap/1 -> -k_G/1
  xgap/1 -> Slipstream reward enable/2, switch2/2, Add1/1
  G1/1 -> switch2/1
  G/1 -> switch2/3
  switch2/1 -> Sum1/3

== system rewardLibrary/Obs // Reward 9-3/Path following ==
  v_err : Inport
  e1 : Inport  Port=2
  e2 : Inport  Port=3
  steer : Inport  Port=4
  accel : Inport  Port=5
  Constant : Constant  Commented=on  Value=0.5
  Exp{,1..4} (5 alike) : Math
  Gain1 : Gain  Gain=0.5
  Gain11 : Gain  Gain=-0.15
  Gain12 : Gain
  Gain2 : Gain  Gain=0.2
  Gain3 : Gain  Gain=0.1
  Gain4 : Gain  Gain=-0.9
  Gain5 : Gain  Gain=-10
  Gain6 : Gain  Gain=1.5
  Gain8 : Gain  Gain=-0.1
  Gain9 : Gain  Gain=-0.06
  Math Function2 : Math  Operator=square  SignedPower=on
  Square{1..4} (4 alike) : Math  Operator=square  SignedPower=on
  Sum1 : Sum  Inputs=++++++
  Unit Delay : UnitDelay  SampleTime=-1  HasFrameUpgradeWarning=on
  Unit Delay1 : UnitDelay  SampleTime=-1  HasFrameUpgradeWarning=on
  r_pf : Outport  VectorParamsAs1DForOutWhenUnconnected=off
  wires:
  Gain11/1 -> Exp/1
  Square4/1 -> Gain11/1
  Exp/1 -> Gain12/1
  v_err/1 -> Square4/1
  Sum1/1 -> r_pf/1
  accel/1 -> Unit Delay1/1
  Square2/1 -> Gain4/1
  steer/1 -> Unit Delay/1
  e1/1 -> Square1/1
  e2/1 -> Square2/1
  Unit Delay/1 -> Math Function2/1  "u_prev"
  Unit Delay1/1 -> Square3/1
  Square3/1 -> Gain8/1
  Math Function2/1 -> Gain5/1
  Square1/1 -> Gain9/1
  Gain8/1 -> Exp4/1
  Gain5/1 -> Exp3/1
  Gain4/1 -> Exp2/1
  Gain9/1 -> Exp1/1
  Exp1/1 -> Gain6/1
  Exp2/1 -> Gain1/1
  Exp3/1 -> Gain2/1
  Exp4/1 -> Gain3/1
  Gain3/1 -> Sum1/5
  Gain2/1 -> Sum1/4
  Gain1/1 -> Sum1/3
  Gain6/1 -> Sum1/2
  Gain12/1 -> Sum1/1
  Constant/1 -> Sum1/6

== system rewardLibrary/Obs // Reward 9-3/Subsystem ==
  v_ego : Inport
  v_ref : Inport  Port=2
  e1 : Inport  Port=3
  e2 : Inport  Port=4
  e1dot : Inport  Port=5
  e2dot : Inport  Port=6
  v_lead : Inport  Port=7
  xgap : Inport  Port=8
  ygap : Inport  Port=9
  Add : Sum  Inputs=+-
  Discrete-Time Integrator1 : DiscreteIntegrator  SampleTime=-1  ICPrevOutput=DiscIntNeverNeededParam  ICPrevScaledInput=DiscIntNeverNeededParam
  Discrete-Time Integrator2 : DiscreteIntegrator  SampleTime=-1  ICPrevOutput=DiscIntNeverNeededParam  ICPrevScaledInput=DiscIntNeverNeededParam
  Discrete-Time Integrator3 : DiscreteIntegrator  SampleTime=-1  ICPrevOutput=DiscIntNeverNeededParam  ICPrevScaledInput=DiscIntNeverNeededParam
  Lateral deviation : Scope
  Mux : Mux  Inputs=12
  obs : Outport  VectorParamsAs1DForOutWhenUnconnected=off
  v_err : Outport  Port=2  VectorParamsAs1DForOutWhenUnconnected=off
  wires:
  ygap/1 -> Mux/12
  xgap/1 -> Mux/11
  v_lead/1 -> Mux/10
  Add/1 -> v_err/1, Mux/2, Discrete-Time Integrator1/1
  Discrete-Time Integrator3/1 -> Mux/6  "integral_error"
  v_ego/1 -> Add/2, Mux/3
  e1/1 -> Lateral deviation/1, Mux/5, Discrete-Time Integrator2/1
  Discrete-Time Integrator1/1 -> Mux/1  "integral_error"
  e2/1 -> Mux/7, Discrete-Time Integrator3/1
  Discrete-Time Integrator2/1 -> Mux/4  "integral_error"
  Mux/1 -> obs/1
  e1dot/1 -> Mux/8
  e2dot/1 -> Mux/9
  v_ref/1 -> Add/1  "d_rel"

== system rewardLibrary/Obs // Reward 9-3/Subsystem2 ==
  v_ego : Inport
  e1 : Inport  Port=2
  e2 : Inport  Port=3
  xgap : Inport  Port=4
  collided : Inport  Port=5
  AND : Logic  IconShape=distinctive  AllPortsSameDT=off  OutDataTypeStr=boolean
  AND1 : Logic  IconShape=distinctive  AllPortsSameDT=off  OutDataTypeStr=boolean
  Abs : Abs  SaturateOnIntegerOverflow=off
  Abs1 : Abs  SaturateOnIntegerOverflow=off
  Compare To Constant : simulink/Logic and Bit Operations/Compare To Constant  relop=>  const=90  OutDataTypeStr=boolean
  Compare To Constant1 : simulink/Logic and Bit Operations/Compare To Constant  relop=>  const=0  OutDataTypeStr=boolean
  Constant : Constant
  Constant3 : Constant  Value=0
  Demux : Demux  Outputs=2
  Detect Rise Positive : simulink/Logic and Bit Operations/Detect Rise Positive  vinit=0  OutDataTypeStr=boolean
  Lateral deviation : simulink/Logic and Bit Operations/Compare To Constant  relop=>  const=8  OutDataTypeStr=boolean
  Logical Operator1 : Logic  Operator=OR  Inputs=3  AllPortsSameDT=off  OutDataTypeStr=boolean
  R2D : Gain  Gain=180/pi
  Relative yaw angle : simulink/Logic and Bit Operations/Compare To Constant  relop=>  const=40  OutDataTypeStr=boolean
  Switch : Switch  Criteria=u2 > Threshold  Threshold=90  SaturateOnIntegerOverflow=off  InputSameDT=off
  Terminator : Terminator
  Velocity : simulink/Logic and Bit Operations/Compare To Constant  relop=<  const=2  OutDataTypeStr=boolean
  Velocity1 : simulink/Logic and Bit Operations/Compare To Constant  relop=<  const=10  OutDataTypeStr=boolean
  fail : Outport  VectorParamsAs1DForOutWhenUnconnected=off
  failCollided : Outport  Port=2  VectorParamsAs1DForOutWhenUnconnected=off
  completeCourse : Outport  Port=3  VectorParamsAs1DForOutWhenUnconnected=off
  overtakeSuccess : Outport  Port=4  VectorParamsAs1DForOutWhenUnconnected=off
  wires:
  collided/1 -> failCollided/1
  AND1/1 -> overtakeSuccess/1
  Compare To Constant1/1 -> AND1/2
  xgap/1 -> Compare To Constant1/1
  Detect Rise Positive/1 -> AND1/1
  Compare To Constant/1 -> Detect Rise Positive/1
  Velocity/1 -> Logical Operator1/1  "tooSlow"
  Lateral deviation/1 -> Logical Operator1/2
  v_ego/1 -> Velocity1/1, Velocity/1
  Abs/1 -> Lateral deviation/1
  e1/1 -> Abs/1
  Velocity1/1 -> AND/1
  e2/1 -> Abs1/1
  Abs1/1 -> R2D/1
  R2D/1 -> Relative yaw angle/1
  Relative yaw angle/1 -> AND/2
  AND/1 -> Logical Operator1/3  "spinTurn"
  Switch/1 -> completeCourse/1
  Constant/1 -> Switch/1
  Constant3/1 -> Switch/3
  Logical Operator1/1 -> fail/1
  Demux/1 -> Terminator/1
  [pos2] -> Demux/1
  Demux/2 -> Switch/2, Compare To Constant/1  "y2"

== system rewardLibrary/Obs // Reward 9-4/Overtaking ==
  note: Overtake on right sigmoid
  note: Overtaking reward sigmoid
  ry : Inport
  xgap : Inport  Port=2
  ygap : Inport  Port=3
  -k_D : Gain  Gain=-0.4
  -k_G : Gain  Gain=-1.2
  Add : Sum
  Add1 : Sum  Inputs=+-
  Add2 : Sum
  C : Gain  Gain=0
  Constant{,2..4} (4 alike) : Constant
  Constant1 : Constant  Value=0
  D : Gain  Gain=9
  Divide : Product  Inputs=*/
  Divide1 : Product  Inputs=*/
  Exp : Math
  Exp1 : Math
  G : Gain  Gain=0.25
  G1 : Constant  Value=0.25
  Memory : Memory
  Slipstream reward enable : Switch  Criteria=u2 > Threshold  Threshold=-6.5  SaturateOnIntegerOverflow=off  InputSameDT=off
  Sum1 : Sum  Inputs=+++
  h : Constant  Value=-2
  switch2 : Switch  Criteria=u2 > Threshold  SaturateOnIntegerOverflow=off  InputSameDT=off
  r_ot : Outport  VectorParamsAs1DForOutWhenUnconnected=off
  wires:
  Constant1/1 -> Slipstream reward enable/1
  C/1 -> Slipstream reward enable/3
  Divide/1 -> D/1
  ry/1 -> C/1
  Slipstream reward enable/1 -> Sum1/1
  Sum1/1 -> r_ot/1
  D/1 -> Sum1/2
  Exp/1 -> Add/1
  Constant/1 -> Divide/1
  -k_D/1 -> Exp/1
  Constant2/1 -> Add/2
  Add/1 -> Divide/2
  Add1/1 -> -k_D/1
  h/1 -> Add1/2
  Constant4/1 -> Add2/2
  Add2/1 -> Divide1/2
  -k_G/1 -> Exp1/1
  Exp1/1 -> Add2/1
  Constant3/1 -> Divide1/1
  Divide1/1 -> G/1
  ygap/1 -> -k_G/1
  xgap/1 -> Slipstream reward enable/2, switch2/2, Add1/1
  G1/1 -> switch2/1
  G/1 -> switch2/3
  switch2/1 -> Sum1/3

== system rewardLibrary/Obs // Reward 9-4/Path following ==
  v_err : Inport
  e1 : Inport  Port=2
  e2 : Inport  Port=3
  steer : Inport  Port=4
  accel : Inport  Port=5
  Constant : Constant  Commented=on  Value=0.5
  Exp{,1..4} (5 alike) : Math
  Gain1 : Gain  Gain=0.5
  Gain11 : Gain  Gain=-0.15
  Gain12 : Gain
  Gain2 : Gain  Gain=0.2
  Gain3 : Gain  Gain=0.1
  Gain4 : Gain  Gain=-0.9
  Gain5 : Gain  Gain=-10
  Gain6 : Gain  Gain=1.5
  Gain8 : Gain  Gain=-0.1
  Gain9 : Gain  Gain=-0.06
  Math Function2 : Math  Operator=square  SignedPower=on
  Square{1..4} (4 alike) : Math  Operator=square  SignedPower=on
  Sum1 : Sum  Inputs=++++++
  Unit Delay : UnitDelay  SampleTime=-1  HasFrameUpgradeWarning=on
  Unit Delay1 : UnitDelay  SampleTime=-1  HasFrameUpgradeWarning=on
  r_pf : Outport  VectorParamsAs1DForOutWhenUnconnected=off
  wires:
  Gain11/1 -> Exp/1
  Square4/1 -> Gain11/1
  Exp/1 -> Gain12/1
  v_err/1 -> Square4/1
  Sum1/1 -> r_pf/1
  accel/1 -> Unit Delay1/1
  Square2/1 -> Gain4/1
  steer/1 -> Unit Delay/1
  e1/1 -> Square1/1
  e2/1 -> Square2/1
  Unit Delay/1 -> Math Function2/1  "u_prev"
  Unit Delay1/1 -> Square3/1
  Square3/1 -> Gain8/1
  Math Function2/1 -> Gain5/1
  Square1/1 -> Gain9/1
  Gain8/1 -> Exp4/1
  Gain5/1 -> Exp3/1
  Gain4/1 -> Exp2/1
  Gain9/1 -> Exp1/1
  Exp1/1 -> Gain6/1
  Exp2/1 -> Gain1/1
  Exp3/1 -> Gain2/1
  Exp4/1 -> Gain3/1
  Gain3/1 -> Sum1/5
  Gain2/1 -> Sum1/4
  Gain1/1 -> Sum1/3
  Gain6/1 -> Sum1/2
  Gain12/1 -> Sum1/1
  Constant/1 -> Sum1/6

== system rewardLibrary/Obs // Reward 9-4/Subsystem ==
  v_ego : Inport
  v_ref : Inport  Port=2
  e1 : Inport  Port=3
  e2 : Inport  Port=4
  e1dot : Inport  Port=5
  e2dot : Inport  Port=6
  v_lead : Inport  Port=7
  xgap : Inport  Port=8
  ygap : Inport  Port=9
  Add : Sum  Inputs=+-
  Discrete-Time Integrator1 : DiscreteIntegrator  SampleTime=-1  ICPrevOutput=DiscIntNeverNeededParam  ICPrevScaledInput=DiscIntNeverNeededParam
  Discrete-Time Integrator2 : DiscreteIntegrator  SampleTime=-1  ICPrevOutput=DiscIntNeverNeededParam  ICPrevScaledInput=DiscIntNeverNeededParam
  Discrete-Time Integrator3 : DiscreteIntegrator  SampleTime=-1  ICPrevOutput=DiscIntNeverNeededParam  ICPrevScaledInput=DiscIntNeverNeededParam
  Lateral deviation : Scope
  Mux : Mux  Inputs=12
  obs : Outport  VectorParamsAs1DForOutWhenUnconnected=off
  v_err : Outport  Port=2  VectorParamsAs1DForOutWhenUnconnected=off
  wires:
  ygap/1 -> Mux/12
  xgap/1 -> Mux/11
  v_lead/1 -> Mux/10
  Add/1 -> v_err/1, Mux/2, Discrete-Time Integrator1/1
  Discrete-Time Integrator3/1 -> Mux/6  "integral_error"
  v_ego/1 -> Add/2, Mux/3
  e1/1 -> Lateral deviation/1, Mux/5, Discrete-Time Integrator2/1
  Discrete-Time Integrator1/1 -> Mux/1  "integral_error"
  e2/1 -> Mux/7, Discrete-Time Integrator3/1
  Discrete-Time Integrator2/1 -> Mux/4  "integral_error"
  Mux/1 -> obs/1
  e1dot/1 -> Mux/8
  e2dot/1 -> Mux/9
  v_ref/1 -> Add/1  "d_rel"

== system rewardLibrary/Obs // Reward 9-4/Subsystem2 ==
  v_ego : Inport
  e1 : Inport  Port=2
  e2 : Inport  Port=3
  xgap : Inport  Port=4
  collided : Inport  Port=5
  AND : Logic  IconShape=distinctive  AllPortsSameDT=off  OutDataTypeStr=boolean
  AND1 : Logic  IconShape=distinctive  AllPortsSameDT=off  OutDataTypeStr=boolean
  Abs : Abs  SaturateOnIntegerOverflow=off
  Abs1 : Abs  SaturateOnIntegerOverflow=off
  Compare To Constant : simulink/Logic and Bit Operations/Compare To Constant  relop=>  const=90  OutDataTypeStr=boolean
  Compare To Constant1 : simulink/Logic and Bit Operations/Compare To Constant  relop=>  const=0  OutDataTypeStr=boolean
  Constant : Constant
  Constant3 : Constant  Value=0
  Demux : Demux  Outputs=2
  Detect Rise Positive : simulink/Logic and Bit Operations/Detect Rise Positive  vinit=0  OutDataTypeStr=boolean
  Lateral deviation : simulink/Logic and Bit Operations/Compare To Constant  relop=>  const=8  OutDataTypeStr=boolean
  Logical Operator1 : Logic  Operator=OR  Inputs=3  AllPortsSameDT=off  OutDataTypeStr=boolean
  R2D : Gain  Gain=180/pi
  Relative yaw angle : simulink/Logic and Bit Operations/Compare To Constant  relop=>  const=30  OutDataTypeStr=boolean
  Switch : Switch  Criteria=u2 > Threshold  Threshold=90  SaturateOnIntegerOverflow=off  InputSameDT=off
  Terminator : Terminator
  Velocity : simulink/Logic and Bit Operations/Compare To Constant  relop=<  const=2  OutDataTypeStr=boolean
  Velocity1 : simulink/Logic and Bit Operations/Compare To Constant  relop=<  const=10  OutDataTypeStr=boolean
  fail : Outport  VectorParamsAs1DForOutWhenUnconnected=off
  failCollided : Outport  Port=2  VectorParamsAs1DForOutWhenUnconnected=off
  completeCourse : Outport  Port=3  VectorParamsAs1DForOutWhenUnconnected=off
  overtakeSuccess : Outport  Port=4  VectorParamsAs1DForOutWhenUnconnected=off
  wires:
  collided/1 -> failCollided/1
  AND1/1 -> overtakeSuccess/1
  Compare To Constant1/1 -> AND1/2
  xgap/1 -> Compare To Constant1/1
  Detect Rise Positive/1 -> AND1/1
  Compare To Constant/1 -> Detect Rise Positive/1
  Velocity/1 -> Logical Operator1/1  "tooSlow"
  Lateral deviation/1 -> Logical Operator1/2
  v_ego/1 -> Velocity1/1, Velocity/1
  Abs/1 -> Lateral deviation/1
  e1/1 -> Abs/1
  Velocity1/1 -> AND/1
  e2/1 -> Abs1/1
  Abs1/1 -> R2D/1
  R2D/1 -> Relative yaw angle/1
  Relative yaw angle/1 -> AND/2
  AND/1 -> Logical Operator1/3  "spinTurn"
  Switch/1 -> completeCourse/1
  Constant/1 -> Switch/1
  Constant3/1 -> Switch/3
  Logical Operator1/1 -> fail/1
  Demux/1 -> Terminator/1
  [pos2] -> Demux/1
  Demux/2 -> Switch/2, Compare To Constant/1  "y2"

== system rewardLibrary/Obs // Reward 9-5/Overtaking ==
  note: Overtake on right sigmoid
  note: Overtaking reward sigmoid
  ry : Inport
  xgap : Inport  Port=2
  ygap : Inport  Port=3
  -k_D : Gain  Gain=-0.4
  -k_G : Gain  Gain=-1.2
  Add : Sum
  Add1 : Sum  Inputs=+-
  Add2 : Sum
  C : Gain  Gain=0
  Constant{,2..4} (4 alike) : Constant
  Constant1 : Constant  Value=0
  D : Gain  Gain=4.25
  Divide : Product  Inputs=*/
  Divide1 : Product  Inputs=*/
  Exp : Math
  Exp1 : Math
  G : Gain  Gain=0.25
  G1 : Constant  Value=0.25
  Slipstream reward enable : Switch  Criteria=u2 > Threshold  Threshold=-6.5  SaturateOnIntegerOverflow=off  InputSameDT=off
  Sum1 : Sum  Inputs=+++
  h : Constant  Value=-2
  switch2 : Switch  Criteria=u2 > Threshold  SaturateOnIntegerOverflow=off  InputSameDT=off
  r_ot : Outport  VectorParamsAs1DForOutWhenUnconnected=off
  wires:
  Constant1/1 -> Slipstream reward enable/1
  C/1 -> Slipstream reward enable/3
  Divide/1 -> D/1
  ry/1 -> C/1
  Slipstream reward enable/1 -> Sum1/1
  Sum1/1 -> r_ot/1
  D/1 -> Sum1/2
  Exp/1 -> Add/1
  Constant/1 -> Divide/1
  -k_D/1 -> Exp/1
  Constant2/1 -> Add/2
  Add/1 -> Divide/2
  Add1/1 -> -k_D/1
  h/1 -> Add1/2
  Constant4/1 -> Add2/2
  Add2/1 -> Divide1/2
  -k_G/1 -> Exp1/1
  Exp1/1 -> Add2/1
  Constant3/1 -> Divide1/1
  Divide1/1 -> G/1
  ygap/1 -> -k_G/1
  xgap/1 -> Slipstream reward enable/2, switch2/2, Add1/1
  G1/1 -> switch2/1
  G/1 -> switch2/3
  switch2/1 -> Sum1/3

== system rewardLibrary/Obs // Reward 9-5/Path following ==
  v_err : Inport
  e1 : Inport  Port=2
  e2 : Inport  Port=3
  steer : Inport  Port=4
  accel : Inport  Port=5
  Constant : Constant  Commented=on  Value=0.5
  Exp{,1..4} (5 alike) : Math
  Gain1 : Gain  Gain=0.5
  Gain11 : Gain  Gain=-0.15
  Gain12 : Gain
  Gain2 : Gain  Gain=0.2
  Gain3 : Gain  Gain=0.1
  Gain4 : Gain  Gain=-0.9
  Gain5 : Gain  Gain=-10
  Gain6 : Gain  Gain=1.5
  Gain8 : Gain  Gain=-0.1
  Gain9 : Gain  Gain=-0.06
  Math Function2 : Math  Operator=square  SignedPower=on
  Square{1..4} (4 alike) : Math  Operator=square  SignedPower=on
  Sum1 : Sum  Inputs=++++++
  Unit Delay : UnitDelay  SampleTime=-1  HasFrameUpgradeWarning=on
  Unit Delay1 : UnitDelay  SampleTime=-1  HasFrameUpgradeWarning=on
  r_pf : Outport  VectorParamsAs1DForOutWhenUnconnected=off
  wires:
  Gain11/1 -> Exp/1
  Square4/1 -> Gain11/1
  Exp/1 -> Gain12/1
  v_err/1 -> Square4/1
  Sum1/1 -> r_pf/1
  accel/1 -> Unit Delay1/1
  Square2/1 -> Gain4/1
  steer/1 -> Unit Delay/1
  e1/1 -> Square1/1
  e2/1 -> Square2/1
  Unit Delay/1 -> Math Function2/1  "u_prev"
  Unit Delay1/1 -> Square3/1
  Square3/1 -> Gain8/1
  Math Function2/1 -> Gain5/1
  Square1/1 -> Gain9/1
  Gain8/1 -> Exp4/1
  Gain5/1 -> Exp3/1
  Gain4/1 -> Exp2/1
  Gain9/1 -> Exp1/1
  Exp1/1 -> Gain6/1
  Exp2/1 -> Gain1/1
  Exp3/1 -> Gain2/1
  Exp4/1 -> Gain3/1
  Gain3/1 -> Sum1/5
  Gain2/1 -> Sum1/4
  Gain1/1 -> Sum1/3
  Gain6/1 -> Sum1/2
  Gain12/1 -> Sum1/1
  Constant/1 -> Sum1/6

== system rewardLibrary/Obs // Reward 9-5/Subsystem ==
  v_ego : Inport
  v_ref : Inport  Port=2
  e1 : Inport  Port=3
  e2 : Inport  Port=4
  e1dot : Inport  Port=5
  e2dot : Inport  Port=6
  v_lead : Inport  Port=7
  xgap : Inport  Port=8
  ygap : Inport  Port=9
  Add : Sum  Inputs=+-
  Discrete-Time Integrator1 : DiscreteIntegrator  SampleTime=-1  ICPrevOutput=DiscIntNeverNeededParam  ICPrevScaledInput=DiscIntNeverNeededParam
  Discrete-Time Integrator2 : DiscreteIntegrator  SampleTime=-1  ICPrevOutput=DiscIntNeverNeededParam  ICPrevScaledInput=DiscIntNeverNeededParam
  Discrete-Time Integrator3 : DiscreteIntegrator  SampleTime=-1  ICPrevOutput=DiscIntNeverNeededParam  ICPrevScaledInput=DiscIntNeverNeededParam
  Lateral deviation : Scope
  Mux : Mux  Inputs=12
  obs : Outport  VectorParamsAs1DForOutWhenUnconnected=off
  v_err : Outport  Port=2  VectorParamsAs1DForOutWhenUnconnected=off
  wires:
  ygap/1 -> Mux/12
  xgap/1 -> Mux/11
  v_lead/1 -> Mux/10
  Add/1 -> v_err/1, Mux/2, Discrete-Time Integrator1/1
  Discrete-Time Integrator3/1 -> Mux/6  "integral_error"
  v_ego/1 -> Add/2, Mux/3
  e1/1 -> Lateral deviation/1, Mux/5, Discrete-Time Integrator2/1
  Discrete-Time Integrator1/1 -> Mux/1  "integral_error"
  e2/1 -> Mux/7, Discrete-Time Integrator3/1
  Discrete-Time Integrator2/1 -> Mux/4  "integral_error"
  Mux/1 -> obs/1
  e1dot/1 -> Mux/8
  e2dot/1 -> Mux/9
  v_ref/1 -> Add/1  "d_rel"

== system rewardLibrary/Obs // Reward 9-5/Subsystem2 ==
  v_ego : Inport
  e1 : Inport  Port=2
  e2 : Inport  Port=3
  xgap : Inport  Port=4
  collided : Inport  Port=5
  AND : Logic  IconShape=distinctive  AllPortsSameDT=off  OutDataTypeStr=boolean
  AND1 : Logic  IconShape=distinctive  AllPortsSameDT=off  OutDataTypeStr=boolean
  Abs : Abs  SaturateOnIntegerOverflow=off
  Abs1 : Abs  SaturateOnIntegerOverflow=off
  Compare To Constant : simulink/Logic and Bit Operations/Compare To Constant  relop=>  const=90  OutDataTypeStr=boolean
  Compare To Constant1 : simulink/Logic and Bit Operations/Compare To Constant  relop=>  const=0  OutDataTypeStr=boolean
  Constant : Constant
  Constant3 : Constant  Value=0
  Demux : Demux  Outputs=2
  Detect Rise Positive : simulink/Logic and Bit Operations/Detect Rise Positive  vinit=0  OutDataTypeStr=boolean
  Lateral deviation : simulink/Logic and Bit Operations/Compare To Constant  relop=>  const=8  OutDataTypeStr=boolean
  Logical Operator1 : Logic  Operator=OR  Inputs=3  AllPortsSameDT=off  OutDataTypeStr=boolean
  R2D : Gain  Gain=180/pi
  Relative yaw angle : simulink/Logic and Bit Operations/Compare To Constant  relop=>  const=40  OutDataTypeStr=boolean
  Switch : Switch  Criteria=u2 > Threshold  Threshold=90  SaturateOnIntegerOverflow=off  InputSameDT=off
  Terminator : Terminator
  Velocity : simulink/Logic and Bit Operations/Compare To Constant  relop=<  const=2  OutDataTypeStr=boolean
  Velocity1 : simulink/Logic and Bit Operations/Compare To Constant  relop=<  const=10  OutDataTypeStr=boolean
  fail : Outport  VectorParamsAs1DForOutWhenUnconnected=off
  failCollided : Outport  Port=2  VectorParamsAs1DForOutWhenUnconnected=off
  completeCourse : Outport  Port=3  VectorParamsAs1DForOutWhenUnconnected=off
  overtakeSuccess : Outport  Port=4  VectorParamsAs1DForOutWhenUnconnected=off
  wires:
  collided/1 -> failCollided/1
  AND1/1 -> overtakeSuccess/1
  Compare To Constant1/1 -> AND1/2
  xgap/1 -> Compare To Constant1/1
  Detect Rise Positive/1 -> AND1/1
  Compare To Constant/1 -> Detect Rise Positive/1
  Velocity/1 -> Logical Operator1/1  "tooSlow"
  Lateral deviation/1 -> Logical Operator1/2
  v_ego/1 -> Velocity1/1, Velocity/1
  Abs/1 -> Lateral deviation/1
  e1/1 -> Abs/1
  Velocity1/1 -> AND/1
  e2/1 -> Abs1/1
  Abs1/1 -> R2D/1
  R2D/1 -> Relative yaw angle/1
  Relative yaw angle/1 -> AND/2
  AND/1 -> Logical Operator1/3  "spinTurn"
  Switch/1 -> completeCourse/1
  Constant/1 -> Switch/1
  Constant3/1 -> Switch/3
  Logical Operator1/1 -> fail/1
  Demux/1 -> Terminator/1
  [pos2] -> Demux/1
  Demux/2 -> Switch/2, Compare To Constant/1  "y2"

== system rewardLibrary/Obs // Reward 9-6/Overtaking ==
  note: Overtake on right sigmoid
  note: Overtaking reward sigmoid
  ry : Inport
  xgap : Inport  Port=2
  ygap : Inport  Port=3
  -k_D : Gain  Gain=-0.3
  -k_G : Gain  Gain=-1.2
  Add : Sum
  Add1 : Sum  Inputs=+-
  Add2 : Sum
  C : Gain  Gain=0
  Constant{,2..4} (4 alike) : Constant
  Constant1 : Constant  Value=0
  D : Gain  Gain=3
  Divide : Product  Inputs=*/
  Divide1 : Product  Inputs=*/
  Exp : Math
  Exp1 : Math
  G : Gain  Gain=0.25
  G1 : Constant  Value=0.25
  Slipstream reward enable : Switch  Criteria=u2 > Threshold  Threshold=-6.5  SaturateOnIntegerOverflow=off  InputSameDT=off
  Sum1 : Sum  Inputs=+++
  h : Constant  Value=-1
  switch2 : Switch  Criteria=u2 > Threshold  SaturateOnIntegerOverflow=off  InputSameDT=off
  r_ot : Outport  VectorParamsAs1DForOutWhenUnconnected=off
  wires:
  Constant1/1 -> Slipstream reward enable/1
  C/1 -> Slipstream reward enable/3
  Divide/1 -> D/1
  ry/1 -> C/1
  Slipstream reward enable/1 -> Sum1/1
  Sum1/1 -> r_ot/1
  D/1 -> Sum1/2
  Exp/1 -> Add/1
  Constant/1 -> Divide/1
  -k_D/1 -> Exp/1
  Constant2/1 -> Add/2
  Add/1 -> Divide/2
  Add1/1 -> -k_D/1
  h/1 -> Add1/2
  Constant4/1 -> Add2/2
  Add2/1 -> Divide1/2
  -k_G/1 -> Exp1/1
  Exp1/1 -> Add2/1
  Constant3/1 -> Divide1/1
  Divide1/1 -> G/1
  ygap/1 -> -k_G/1
  xgap/1 -> Slipstream reward enable/2, switch2/2, Add1/1
  G1/1 -> switch2/1
  G/1 -> switch2/3
  switch2/1 -> Sum1/3
